simulink model "VISUAL_DisturbanceRejection"  (R2022a)
settings: Solver=VariableStepAuto  StartTime=0.0  StopTime=10.0  RelTol=1e-3
settings Model: Creator=feyzi  LastModifiedBy=feyzi

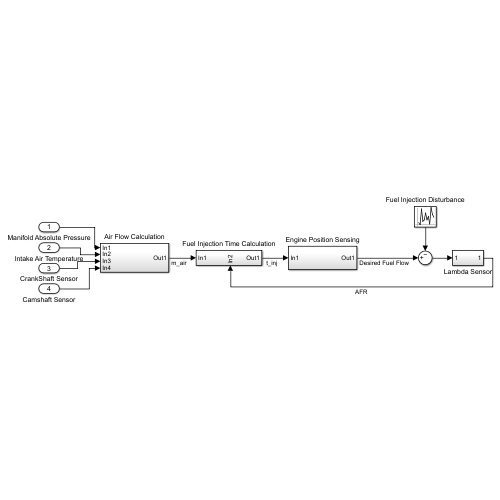
[thumbnail: Simulink's stored preview of the top-level diagram]
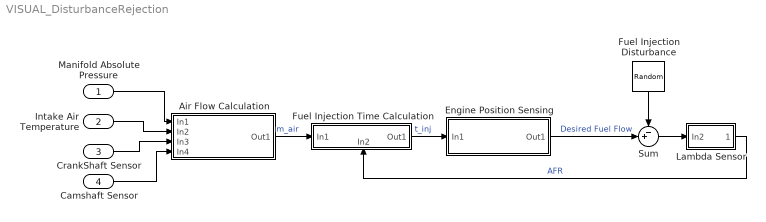
== system VISUAL_DisturbanceRejection ==
  Manifold Absolute Pressure : Inport
  Intake Air Temperature : Inport  Port=2
  CrankShaft Sensor : Inport  Port=3
  Camshaft Sensor : Inport  Port=4
  Air Flow Calculation : Subsystem
  Engine Position Sensing : Subsystem
  Fuel Injection Disturbance : UniformRandomNumber  SampleTime=0.1
  Fuel Injection Time Calculation : Subsystem
      settings: PortSchema="{\"entries\":[{\"content\":{\"sides\":[{\"content\":{\"connectorIds\":[\"In1\"]},\"type\":\"ConnectorPlacement.EquallySpacedRectSide\",\"uuid\":\"ea5dcee3-032b-4474-bae9-82d0a9206779\"},{\"content\":{\"connectorIds\":[\"Out1\"],\"side\":\"RIGHT\"},\"type\":\"ConnectorPlacement.EquallySpacedRectSide\",\"uuid\":\"25a77294-0096-4cf3-a4c7-02c9e7eb2602\"},{\"content\":{\"connectorIds\":[],\"side\":\"TOP\"},\"type\":\"ConnectorPlacement.EquallySpacedRectSide\",\"uuid\":\"609e78f2-0ac6-480f-a8f3-5ca01ce85e2f\"},{\"content\":{\"connectorIds\":[\"In2\"],\"side\":\"BOTTOM\"},\"type\":\"ConnectorPlacement.EquallySpacedRectSide\",\"uuid\":\"2866d651-891c-4862-a3c3-9ef9e638504c\"}]},\"type\":\"ConnectorPlacement.EquallySpacedConnector\",\"uuid\":\"eb0256f2-4870-42fc-9cd8-82e32e4fb826\"}],\"packageUris\":[\"http://schema.mathworks.com/mf0/Connector/R2020b\"],\"version\":\"1.0\"}"
  Lambda Sensor : Subsystem
  Sum : Sum  Inputs=-+|
  wires:
  Manifold Absolute Pressure/1 -> Air Flow Calculation/1(In1)
  Air Flow Calculation/1(Out1) -> Fuel Injection Time Calculation/1(In1)  "m_air"
  Lambda Sensor/1(Out1) -> Fuel Injection Time Calculation/2(In2)  "AFR"
  CrankShaft Sensor/1 -> Air Flow Calculation/3(In3)
  Fuel Injection Time Calculation/1(Out1) -> Engine Position Sensing/1(In1)  "t_inj"
  Engine Position Sensing/1(Out1) -> Sum/2  "Desired Fuel Flow"
  Fuel Injection Disturbance/1 -> Sum/1
  Sum/1 -> Lambda Sensor/1(In2)
  Intake Air Temperature/1 -> Air Flow Calculation/2(In2)
  Camshaft Sensor/1 -> Air Flow Calculation/4(In4)

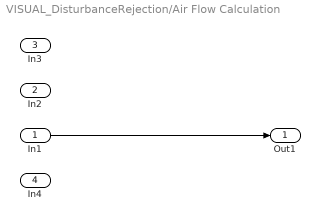
== system VISUAL_DisturbanceRejection/Air Flow Calculation ==
  In1 : Inport
  In2 : Inport  Port=2
  In3 : Inport  Port=3
  In4 : Inport  Port=4
  Out1 : Outport
  wires:
  In1/1 -> Out1/1

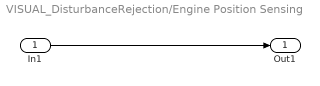
== system VISUAL_DisturbanceRejection/Engine Position Sensing ==
  In1 : Inport
  Out1 : Outport
  wires:
  In1/1 -> Out1/1

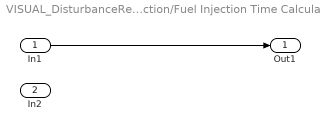
== system VISUAL_DisturbanceRejection/Fuel Injection Time Calculation ==
  In1 : Inport
  In2 : Inport  Port=2
  Out1 : Outport
  wires:
  In1/1 -> Out1/1

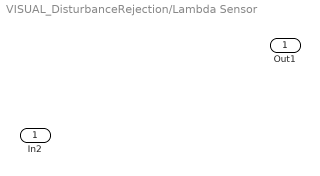
== system VISUAL_DisturbanceRejection/Lambda Sensor ==
  In2 : Inport
  Out1 : Outport
  wires:
  ? -> Out1/1
